simulink model "MRly_VD"  (R2016b)
settings: configuration reference "CodeGenConfigSet" (kept outside this file)
values from neighbouring files (symbols this model uses):
  MRly_ctErlyOpng_C = Calibration.Parameter    [init_MRly_VD.m]
  MRly_facBattVltgFlt_C = Calibration.Parameter    [init_MRly_VD.m]
  MRly_tiCloseStk_C = Calibration.Parameter    [init_MRly_VD.m]
  MRly_tiStkRlyDiaDel_C = Calibration.Parameter    [init_MRly_VD.m]
  MRly_uStkRlyBattThr_C = Calibration.Parameter    [init_MRly_VD.m]
undefined symbols (not defined in the file or in its folder): MRly_VD_DT
libraries: CXLib x9
settings Model: Creator=Administrator  LastModifiedBy=lenovo
settings ConfigSetRef: SourceLocation=Base Workspace

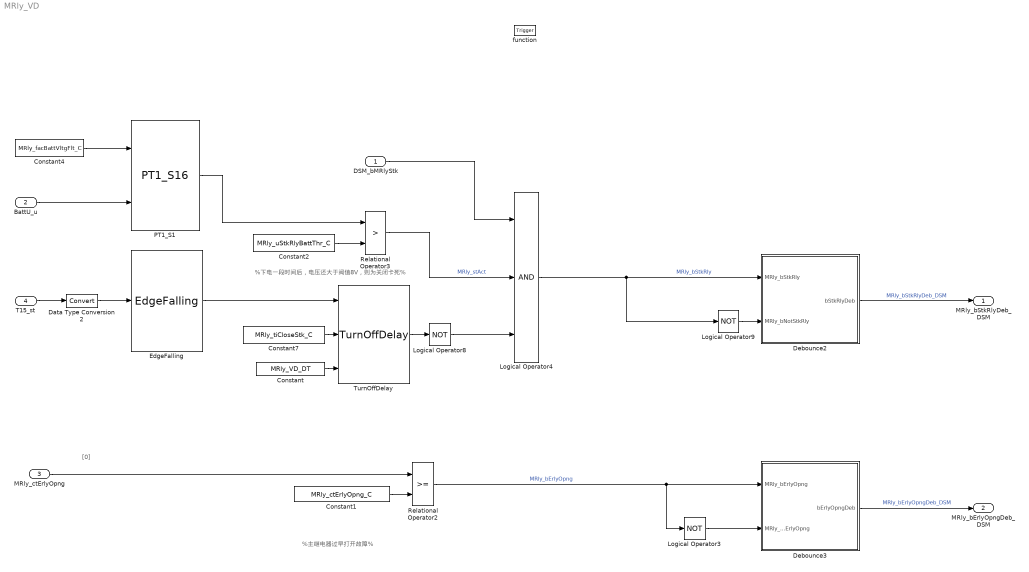
== system MRly_VD ==
  note: [0]
  note: %主继电器过早打开故障%
  note: %下电一段时间后，电压还大于阀值8V，则为关闭卡死%
  DSM_bMRlyStk : Inport  Description=state of Fid_MRlyStk  OutMin=0  OutMax=1  OutDataTypeStr=boolean
  BattU_u : Inport  Tag=mv  Description=Battery voltage  Port=2  OutMin=0  OutMax=50000  OutDataTypeStr=Battery_mv
  MRly_ctErlyOpng : Inport  Description=Errorcounter-message to detect early opening of the main relay  Port=3  OutMin=0  OutMax=255  OutDataTypeStr=Counter_num
  T15_st : Inport  Description=Terminal 15 status after debouncing  Port=4  OutDataTypeStr=Enum: Switch_conv
  function : TriggerPort  TriggerType=function-call  VariantControl=Variant
  Constant : Constant  Value=MRly_VD_DT
  Constant1 : Constant  Value=MRly_ctErlyOpng_C  SampleTime=-1
  Constant2 : Constant  Value=MRly_uStkRlyBattThr_C  SampleTime=-1
  Constant4 : Constant  Value=MRly_facBattVltgFlt_C  SampleTime=-1
  Constant7 : Constant  Value=MRly_tiCloseStk_C  SampleTime=-1
  Data Type Conversion2 : DataTypeConversion
  Debounce2 : Subsystem
  Debounce3 : Subsystem
  EdgeFalling : CXLib/EdgeFalling
  Logical Operator3 : Logic  Operator=NOT  AllPortsSameDT=off  OutDataTypeStr=boolean
  Logical Operator4 : Logic  Inputs=3  OutDataTypeStr=boolean
  Logical Operator8 : Logic  Operator=NOT  AllPortsSameDT=off  OutDataTypeStr=boolean
  Logical Operator9 : Logic  Operator=NOT  AllPortsSameDT=off  OutDataTypeStr=boolean
  PT1_S1 : CXLib/PT1_S16
  Relational Operator2 : RelationalOperator  OutDataTypeStr=boolean  RndMeth=Nearest  InputSameDT=on
  Relational Operator3 : RelationalOperator  Operator=>  OutDataTypeStr=boolean  RndMeth=Nearest  InputSameDT=on
  TurnOffDelay : CXLib/TurnOffDelay
  MRly_bStkRlyDeb_DSM : Outport  Description=To prevent the jammed  OutMin=0  OutMax=1  OutDataTypeStr=boolean
  MRly_bErlyOpngDeb_DSM : Outport  Description=Prevent premature opening  Port=2  OutMin=0  OutMax=1  OutDataTypeStr=boolean
  wires:
  Constant1/1 -> Relational Operator2/2
  MRly_ctErlyOpng/1 -> Relational Operator2/1
  BattU_u/1 -> PT1_S1/2
  Constant2/1 -> Relational Operator3/2
  DSM_bMRlyStk/1 -> Logical Operator4/1
  Relational Operator3/1 -> Logical Operator4/2  "MRly_stAct"
  PT1_S1/1 -> Relational Operator3/1
  Constant4/1 -> PT1_S1/1
  Debounce2/1(bStkRlyDeb) -> MRly_bStkRlyDeb_DSM/1  "MRly_bStkRlyDeb_DSM"
  Logical Operator4/1 -> Debounce2/1(MRly_bStkRly), Logical Operator9/1  "MRly_bStkRly"
  Logical Operator9/1 -> Debounce2/2(MRly_bNotStkRly)
  Debounce3/1(bErlyOpngDeb) -> MRly_bErlyOpngDeb_DSM/1  "MRly_bErlyOpngDeb_DSM"
  Relational Operator2/1 -> Logical Operator3/1, Debounce3/1(MRly_bErlyOpng)  "MRly_bErlyOpng"
  Logical Operator3/1 -> Debounce3/2(MRly_bNotErlyOpng)
  Data Type Conversion2/1 -> EdgeFalling/1
  Constant7/1 -> TurnOffDelay/2
  Constant/1 -> TurnOffDelay/3
  TurnOffDelay/1 -> Logical Operator8/1
  EdgeFalling/1 -> TurnOffDelay/1
  Logical Operator8/1 -> Logical Operator4/3
  T15_st/1 -> Data Type Conversion2/1

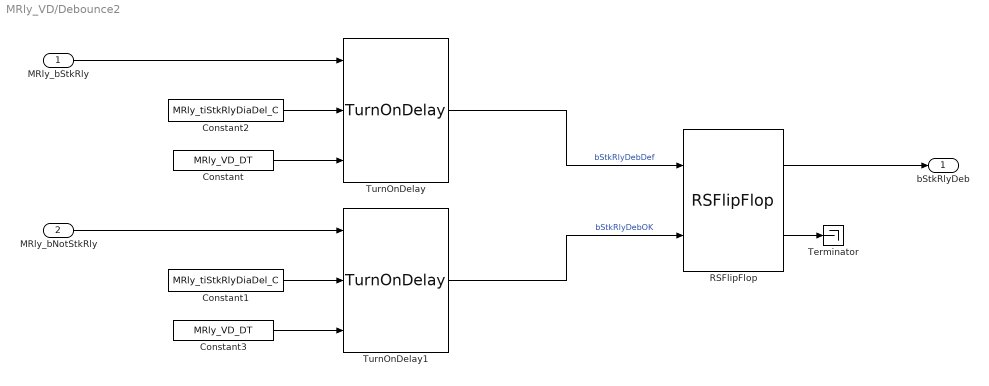
== system MRly_VD/Debounce2 ==
  MRly_bStkRly : Inport
  MRly_bNotStkRly : Inport  Port=2
  Constant : Constant  Value=MRly_VD_DT
  Constant1 : Constant  Value=MRly_tiStkRlyDiaDel_C
  Constant2 : Constant  Value=MRly_tiStkRlyDiaDel_C
  Constant3 : Constant  Value=MRly_VD_DT
  RSFlipFlop : CXLib/RSFlipFlop
  Terminator : Terminator
  TurnOnDelay : CXLib/TurnOnDelay
  TurnOnDelay1 : CXLib/TurnOnDelay
  bStkRlyDeb : Outport
  wires:
  RSFlipFlop/1 -> bStkRlyDeb/1
  TurnOnDelay1/1 -> RSFlipFlop/2  "bStkRlyDebOK"
  Constant1/1 -> TurnOnDelay1/2
  Constant2/1 -> TurnOnDelay/2
  TurnOnDelay/1 -> RSFlipFlop/1  "bStkRlyDebDef"
  MRly_bNotStkRly/1 -> TurnOnDelay1/1
  RSFlipFlop/2 -> Terminator/1
  MRly_bStkRly/1 -> TurnOnDelay/1
  Constant/1 -> TurnOnDelay/3
  Constant3/1 -> TurnOnDelay1/3

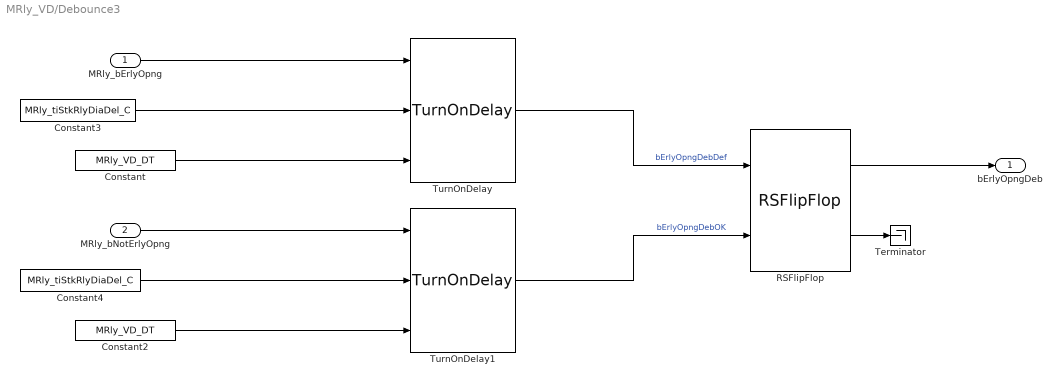
== system MRly_VD/Debounce3 ==
  MRly_bErlyOpng : Inport
  MRly_bNotErlyOpng : Inport  Port=2
  Constant : Constant  Value=MRly_VD_DT
  Constant2 : Constant  Value=MRly_VD_DT
  Constant3 : Constant  Value=MRly_tiStkRlyDiaDel_C
  Constant4 : Constant  Value=MRly_tiStkRlyDiaDel_C
  RSFlipFlop : CXLib/RSFlipFlop
  Terminator : Terminator
  TurnOnDelay : CXLib/TurnOnDelay
  TurnOnDelay1 : CXLib/TurnOnDelay
  bErlyOpngDeb : Outport
  wires:
  MRly_bErlyOpng/1 -> TurnOnDelay/1
  RSFlipFlop/2 -> Terminator/1
  MRly_bNotErlyOpng/1 -> TurnOnDelay1/1
  TurnOnDelay/1 -> RSFlipFlop/1  "bErlyOpngDebDef"
  Constant3/1 -> TurnOnDelay/2
  Constant4/1 -> TurnOnDelay1/2
  TurnOnDelay1/1 -> RSFlipFlop/2  "bErlyOpngDebOK"
  RSFlipFlop/1 -> bErlyOpngDeb/1
  Constant/1 -> TurnOnDelay/3
  Constant2/1 -> TurnOnDelay1/3
